simulink library "lib_wheel2"  (Simulink 10.1)
settings: Solver=VariableStepAuto  StartTime=0.0  StopTime=10.0  RelTol=1e-3
undefined symbols (not defined in the file or in its folder): lib_help, NOTES, veh_air_density, veh_CD, veh_cg_height, veh_FA, veh_front_wt_frac, veh_gravity, veh_roadwheel_radius, veh_rr_a, veh_rr_alpha, veh_rr_b, veh_rr_beta, veh_rr_c, veh_wheelbase, wh_1st_rrc, wh_2nd_rrc, wh_axle_loss_mass, wh_axle_loss_trq, wh_fa_dl_brake_frac, wh_fa_dl_brake_mph, wh_fa_fric_brake_frac, wh_fa_fric_brake_mph, wh_front_active_bool, wh_inertia, wh_max_front_brake_force, wh_max_rear_brake_force, wh_pressure, wh_radius, wh_rear_active_bool, wh_slip, wh_slip_force_coeff
undefined symbols (not defined in the file): logFlag
libraries: $bdroot x61, lib_vehicle x2, lib_etc x2, lib_controls x2, lib_wheel x1
(part 13 of 13)

== system lib_wheel2/development/wheel and axle  front/rear <wh> 2 axle --> 1 driveline/wheel & axle model & interface/wheel model/tire slip model (m/s) ==
  note: See note regarding sum in backward path
  weight borne  by front axle (N) : Inport
  total tractive  force available (N) : Inport  Port=2
  axle speed available (rad/s) : Inport  Port=3
  axle speed req'd (rad/s) : Inport  Port=4
  vehicle speed required (m/s) : Inport  Port=5
  weight borne by  rear axle (N) : Inport  Port=6
  front fraction : Inport  Port=7
  Abs1 : Abs  SaturateOnIntegerOverflow=on
  Block NOTES : Subsystem
      mask Display: disp('Block\nNOTES')
  Constant : Constant  Value=1e-3
  Constant5 : Constant
  Constant6 : Constant  Value=wh_radius
  Fcn : Fcn  Expr=1/u
  Relational Operator1 : RelationalOperator  Operator=>  RndMeth=Nearest  InputSameDT=on
  Sum1 : Sum  Inputs=+-  SaturateOnIntegerOverflow=on
  Sum2 : Sum  SaturateOnIntegerOverflow=on
  Sum3 : Sum  SaturateOnIntegerOverflow=on
  Sum4 : Sum  Inputs=-+  SaturateOnIntegerOverflow=on
  Switch1 : Switch  Threshold=eps  SaturateOnIntegerOverflow=on  InputSameDT=on
  front axle : Subsystem
  front frac : Product  SaturateOnIntegerOverflow=on
  rear axle : Subsystem
  vehicle speed (m/s) : Product  Inputs=3  SaturateOnIntegerOverflow=on
  possible vehicle speed (m/s) : Outport  InitialOutput=0
  tag scope: veh_spd_a_rec=global
  wires:
  Sum3/1 -> Fcn/1
  Fcn/1 -> vehicle speed (m/s)/1
  Constant5/1 -> Sum3/2
  axle speed available (rad/s)/1 -> Sum4/1, vehicle speed (m/s)/2
  Constant6/1 -> vehicle speed (m/s)/3
  Relational Operator1/1 -> Switch1/2
  vehicle speed required (m/s)/1 -> Switch1/3
  Sum4/1 -> Abs1/1
  axle speed req'd (rad/s)/1 -> Sum4/2
  Constant/1 -> Relational Operator1/2
  Abs1/1 -> Relational Operator1/1
  weight borne  by front axle (N)/1 -> front axle/1(In1)
  Switch1/1 -> possible vehicle speed (m/s)/1
  vehicle speed (m/s)/1 -> Switch1/1, [veh_spd_a_rec]
  weight borne by  rear axle (N)/1 -> rear axle/1(In1)
  total tractive  force available (N)/1 -> front frac/1, Sum1/1
  front fraction/1 -> front frac/2
  front frac/1 -> front axle/2(In2), Sum1/2
  Sum1/1 -> rear axle/2(In2)
  front axle/1(Out1) -> Sum2/1
  rear axle/1(Out1) -> Sum2/2
  Sum2/1 -> Sum3/1

== system lib_wheel2/development/wheel and axle  front/rear <wh> 2 axle --> 1 driveline/wheel & axle model & interface/wheel model/tire slip model (rad/s) ==
  note: Slip is defined as s=(omega*r - v) / v.  The one-to-one mapping of slip to normalized
      | tractive force, F_tract/W_front_axle, up to the maximum, is stored in the variables
      | "wh_slip" and "wh_slip_force_coeff."
  note: This block implements the effects of finite tire slip
      | (with respect to the road) on the vehicle speed/wheel speed relationship.
  note: Question: for front and rear, is it the sum of or min/max? tm:020703
  total tractive  force requested (N) : Inport
  requested time-step average vehicle speed (m/s) : Inport  Port=2
  weight borne by front axle (N) : Inport  Port=3
  weight borne by  rear axle (N)1 : Inport  Port=4
  front traction ratio : Inport  Port=5
  Constant5 : Constant
  Constant6 : Constant  Value=1/wh_radius
  Sum1 : Sum  Inputs=+-  SaturateOnIntegerOverflow=on
  Sum2 : Sum  SaturateOnIntegerOverflow=on
  Sum3 : Sum  SaturateOnIntegerOverflow=on
  To Workspace6 : ToWorkspace  VariableName=wh_slip_r  SampleTime=-1
  front frac : Product  SaturateOnIntegerOverflow=on
  front slip : Subsystem
  rear slip : Subsystem
  wheel speed (rad/s) : Product  Inputs=3  SaturateOnIntegerOverflow=on
  slip-augmented rotational speed (rad/s) : Outport  InitialOutput=0
  wires:
  weight borne by front axle (N)/1 -> front slip/1(In1)
  requested time-step average vehicle speed (m/s)/1 -> wheel speed (rad/s)/1
  Constant6/1 -> wheel speed (rad/s)/3
  Sum3/1 -> wheel speed (rad/s)/2
  Constant5/1 -> Sum3/2
  wheel speed (rad/s)/1 -> slip-augmented rotational speed (rad/s)/1
  front frac/1 -> Sum1/2, front slip/2(In2)
  total tractive  force requested (N)/1 -> front frac/1, Sum1/1
  front traction ratio/1 -> front frac/2
  Sum1/1 -> rear slip/2(In2)
  weight borne by  rear axle (N)1/1 -> rear slip/1(In1)
  front slip/1(Out1) -> Sum2/1
  rear slip/1(Out1) -> Sum2/2
  Sum2/1 -> Sum3/1, To Workspace6/1

== system lib_wheel2/development/wheel and axle  front/rear <wh> 2 axle --> 1 driveline/wheel & axle model & interface/wheel model/traction controller interface ==
  F_req : Inport
  v_ave_req : Inport  Port=2
  F_req_limited : Outport  InitialOutput=0
  v_req_limited : Outport  Port=2  InitialOutput=0
  wt_front_axle : Outport  Port=3  InitialOutput=0
  wt_rear_axle : Outport  Port=4  InitialOutput=0
  front_traction_ratio : Outport  Port=5  InitialOutput=0
  tag scope: F_req=global, v_ave_req=global
  wires:
  [F_req_limited] -> F_req_limited/1
  [v_req_limited] -> v_req_limited/1
  [wt_front_axle] -> wt_front_axle/1
  F_req/1 -> [F_req]
  v_ave_req/1 -> [v_ave_req]
  [wt_rear_axle] -> wt_rear_axle/1
  [front_traction_ratio] -> front_traction_ratio/1

== system lib_wheel2/vehicle, wheel, & axle front/rear <wh>/models and interface/vehicle <veh>/record achieved force outputs/enhancedToWorkspace ==
  In1 : Inport
  To Workspace : ToWorkspace  VariableName=veh_pwr_accel_a  SampleTime=-1
  wires:
  In1/1 -> To Workspace/1

== system lib_wheel2/vehicle, wheel, & axle front/rear <wh>/models and interface/vehicle <veh>/record achieved force outputs/enhancedToWorkspace1 ==
  In1 : Inport
  To Workspace : ToWorkspace  VariableName=veh_pwr_drag_a  SampleTime=-1
  wires:
  In1/1 -> To Workspace/1

== system lib_wheel2/vehicle, wheel, & axle front/rear <wh>/models and interface/vehicle <veh>/record achieved force outputs/enhancedToWorkspace2 ==
  In1 : Inport
  To Workspace : ToWorkspace  VariableName=veh_pwr_ascent_a  SampleTime=-1
  wires:
  In1/1 -> To Workspace/1

== system lib_wheel2/vehicle, wheel, & axle front/rear <wh>/models and interface/vehicle <veh>/record achieved force outputs/enhancedToWorkspace3 ==
  In1 : Inport
  To Workspace : ToWorkspace  VariableName=veh_pwr_rr_a  SampleTime=-1
  wires:
  In1/1 -> To Workspace/1

== system lib_wheel2/vehicle, wheel, & axle front/rear <wh>/models and interface/vehicle <veh>/record achieved force outputs/rolling resistance force ==
  average vehicle speed over time step (m/s) : Inport
  force req'd to overcome rolling resistance (N) : $bdroot/Submodels/force req'd to overcome rolling resistance (N)
      settings: RTWFcnNameOpts=Auto  RTWFileNameOpts=Auto
  Fr (N) : Outport
  wires:
  average vehicle speed over time step (m/s)/1 -> force req'd to overcome rolling resistance (N)/1
  force req'd to overcome rolling resistance (N)/1 -> Fr (N)/1

== system lib_wheel2/vehicle, wheel, & axle front/rear <wh>/models and interface/wheel and axle  front/rear <wh>/front force/brake request  controller interface ==
  F_front_brake_req : Outport  InitialOutput=0
  wires:
  [F_front_brake_req] -> F_front_brake_req/1

== system lib_wheel2/vehicle, wheel, & axle front/rear <wh>/models and interface/wheel and axle  front/rear <wh>/front force/enhancedToWorkspace11 ==
  In1 : Inport
  To Workspace : ToWorkspace  VariableName=wh_front_brake_r  SampleTime=-1
  wires:
  In1/1 -> To Workspace/1

== system lib_wheel2/vehicle, wheel, & axle front/rear <wh>/models and interface/wheel and axle  front/rear <wh>/limits and losses diagnostics/enhancedToWorkspace ==
  In1 : Inport
  To Workspace : ToWorkspace  VariableName=wh_brake_loss_pwr  SampleTime=-1
  wires:
  In1/1 -> To Workspace/1

== system lib_wheel2/vehicle, wheel, & axle front/rear <wh>/models and interface/wheel and axle  front/rear <wh>/rear force/brake request controller interface1 ==
  F_rear_brake_req : Outport  InitialOutput=0
  wires:
  [F_rear_brake_req] -> F_rear_brake_req/1

== system lib_wheel2/vehicle, wheel, & axle front/rear <wh>/models and interface/wheel and axle  front/rear <wh>/rear force/enhancedToWorkspace ==
  In1 : Inport
  To Workspace : ToWorkspace  VariableName=wh_rear_brake_r  SampleTime=-1
  wires:
  In1/1 -> To Workspace/1

== system lib_wheel2/vehicle, wheel, & axle front/rear <wh>/models and interface/wheel and axle  front/rear <wh>/tire slip model (m/s)/Block NOTES ==
  note: This block implements the effects of finite tire slip (with respect to the road) on the
      | vehicle speed/wheel speed relationship.  Slip is defined as s=(omega*r - v) / v.  The
      | one-to-one mapping of slip to normalized tractive force, F_tract/W_front_axle, up to
      | the maximum, is stored in the variables "wh_slip" and "wh_slip_force_coeff."  The
      | slip calculation here is overridden if the actual axle speed and the requested axle
      | speed are the same, indicating that no drivetrain speed limits were encountered.

== system lib_wheel2/vehicle, wheel, & axle front/rear <wh>/models and interface/wheel and axle  front/rear <wh>/tire slip model (m/s)/front axle ==
  In1 : Inport
  In2 : Inport  Port=2
  Abs : Abs  SaturateOnIntegerOverflow=on
  Constant3 : Constant  Value=0
  F/W : Product  Inputs=*/  SaturateOnIntegerOverflow=on
  Product : Product  SaturateOnIntegerOverflow=on
  Relational Operator : RelationalOperator  Operator=~=  RndMeth=Nearest  InputSameDT=on
  Saturation : Saturate  UpperLimit=max(wh_slip_force_coeff)  LowerLimit=min(wh_slip_force_coeff)
  Sign : Signum
  Switch : Switch  SaturateOnIntegerOverflow=on  InputSameDT=on
  s=s(F/W) : Lookup  InputValues=wh_slip_force_coeff  Table=wh_slip  SaturateOnIntegerOverflow=on
  Out1 : Outport
  wires:
  Constant3/1 -> Switch/3, Relational Operator/2
  Relational Operator/1 -> Switch/2
  Abs/1 -> F/W/1, Relational Operator/1
  Saturation/1 -> s=s(F/W)/1
  Switch/1 -> Saturation/1
  F/W/1 -> Switch/1
  Sign/1 -> Product/2
  s=s(F/W)/1 -> Product/1
  In2/1 -> Abs/1, Sign/1
  In1/1 -> F/W/2
  Product/1 -> Out1/1

== system lib_wheel2/vehicle, wheel, & axle front/rear <wh>/models and interface/wheel and axle  front/rear <wh>/tire slip model (m/s)/rear axle ==
  In1 : Inport
  In2 : Inport  Port=2
  Abs : Abs  SaturateOnIntegerOverflow=on
  Constant3 : Constant  Value=0
  F/W : Product  Inputs=*/  SaturateOnIntegerOverflow=on
  Product : Product  SaturateOnIntegerOverflow=on
  Relational Operator : RelationalOperator  Operator=~=  RndMeth=Nearest  InputSameDT=on
  Saturation : Saturate  UpperLimit=max(wh_slip_force_coeff)  LowerLimit=min(wh_slip_force_coeff)
  Sign : Signum
  Switch : Switch  SaturateOnIntegerOverflow=on  InputSameDT=on
  s=s(F/W) : Lookup  InputValues=wh_slip_force_coeff  Table=wh_slip  SaturateOnIntegerOverflow=on
  Out1 : Outport
  wires:
  Constant3/1 -> Switch/3, Relational Operator/2
  Relational Operator/1 -> Switch/2
  Abs/1 -> F/W/1, Relational Operator/1
  Saturation/1 -> s=s(F/W)/1
  Switch/1 -> Saturation/1
  F/W/1 -> Switch/1
  Sign/1 -> Product/2
  s=s(F/W)/1 -> Product/1
  In2/1 -> Abs/1, Sign/1
  In1/1 -> F/W/2
  Product/1 -> Out1/1

== system lib_wheel2/vehicle, wheel, & axle front/rear <wh>/models and interface/wheel and axle  front/rear <wh>/tire slip model (rad/s)/enhancedToWorkspace ==
  In1 : Inport
  To Workspace : ToWorkspace  VariableName=wh_slip_r  SampleTime=-1
  wires:
  In1/1 -> To Workspace/1

== system lib_wheel2/vehicle, wheel, & axle front/rear <wh>/models and interface/wheel and axle  front/rear <wh>/tire slip model (rad/s)/front slip ==
  In1 : Inport
  In2 : Inport  Port=2
  Abs : Abs  SaturateOnIntegerOverflow=on
  F/W : Product  Inputs=*/  SaturateOnIntegerOverflow=on
  Product : Product  SaturateOnIntegerOverflow=on
  Saturation : Saturate  UpperLimit=max(wh_slip_force_coeff)  LowerLimit=min(wh_slip_force_coeff)
  Sign : Signum
  s=s(F/W) : Lookup  InputValues=wh_slip_force_coeff  Table=wh_slip  SaturateOnIntegerOverflow=on
  Out1 : Outport
  wires:
  Saturation/1 -> s=s(F/W)/1
  F/W/1 -> Saturation/1
  Abs/1 -> F/W/1
  Sign/1 -> Product/2
  In2/1 -> Abs/1, Sign/1
  s=s(F/W)/1 -> Product/1
  In1/1 -> F/W/2
  Product/1 -> Out1/1

== system lib_wheel2/vehicle, wheel, & axle front/rear <wh>/models and interface/wheel and axle  front/rear <wh>/tire slip model (rad/s)/rear slip ==
  In1 : Inport
  In2 : Inport  Port=2
  Abs : Abs  SaturateOnIntegerOverflow=on
  F/W : Product  Inputs=*/  SaturateOnIntegerOverflow=on
  Product : Product  SaturateOnIntegerOverflow=on
  Saturation : Saturate  UpperLimit=max(wh_slip_force_coeff)  LowerLimit=min(wh_slip_force_coeff)
  Sign : Signum
  s=s(F/W) : Lookup  InputValues=wh_slip_force_coeff  Table=wh_slip  SaturateOnIntegerOverflow=on
  Out1 : Outport
  wires:
  Saturation/1 -> s=s(F/W)/1
  F/W/1 -> Saturation/1
  Abs/1 -> F/W/1
  Sign/1 -> Product/2
  In2/1 -> Abs/1, Sign/1
  s=s(F/W)/1 -> Product/1
  In1/1 -> F/W/2
  Product/1 -> Out1/1

== system lib_wheel2/vehicle, wheel, & axle front/rear <wh> 2 axle --> 1 driveline/models and interface/vehicle <veh>/power logging--achieved/Joules ==
  In1 : Inport
  To Workspace : ToWorkspace  VariableName=veh_energy_a  SampleTime=-1
  wires:
  In1/1 -> To Workspace/1

== system lib_wheel2/vehicle, wheel, & axle front/rear <wh> 2 axle --> 1 driveline/models and interface/vehicle <veh>/power logging--achieved/horse power ==
  In1 : Inport
  To Workspace : ToWorkspace  VariableName=veh_pwr_a_hp  SampleTime=-1
  wires:
  In1/1 -> To Workspace/1

== system lib_wheel2/vehicle, wheel, & axle front/rear <wh> 2 axle --> 1 driveline/models and interface/vehicle <veh>/power logging--achieved/watts ==
  In1 : Inport
  To Workspace : ToWorkspace  VariableName=veh_pwr_a  SampleTime=-1
  wires:
  In1/1 -> To Workspace/1

== system lib_wheel2/vehicle, wheel, & axle front/rear <wh> 2 axle --> 1 driveline/models and interface/vehicle <veh>/power logging--request/Joules ==
  In1 : Inport
  To Workspace : ToWorkspace  VariableName=veh_energy_r  SampleTime=-1
  wires:
  In1/1 -> To Workspace/1

== system lib_wheel2/vehicle, wheel, & axle front/rear <wh> 2 axle --> 1 driveline/models and interface/vehicle <veh>/power logging--request/horse power ==
  In1 : Inport
  To Workspace : ToWorkspace  VariableName=veh_pwr_r_hp  SampleTime=-1
  wires:
  In1/1 -> To Workspace/1

== system lib_wheel2/vehicle, wheel, & axle front/rear <wh> 2 axle --> 1 driveline/models and interface/vehicle <veh>/power logging--request/watts ==
  In1 : Inport
  To Workspace : ToWorkspace  VariableName=veh_pwr_r  SampleTime=-1
  wires:
  In1/1 -> To Workspace/1

== system lib_wheel2/vehicle, wheel, & axle front/rear <wh> 2 axle --> 1 driveline/models and interface/vehicle <veh>/record achieved force outputs/enhancedToWorkspace ==
  In1 : Inport
  To Workspace : ToWorkspace  VariableName=veh_pwr_accel_a  SampleTime=-1
  wires:
  In1/1 -> To Workspace/1

== system lib_wheel2/vehicle, wheel, & axle front/rear <wh> 2 axle --> 1 driveline/models and interface/vehicle <veh>/record achieved force outputs/enhancedToWorkspace1 ==
  In1 : Inport
  To Workspace : ToWorkspace  VariableName=veh_pwr_drag_a  SampleTime=-1
  wires:
  In1/1 -> To Workspace/1

== system lib_wheel2/vehicle, wheel, & axle front/rear <wh> 2 axle --> 1 driveline/models and interface/vehicle <veh>/record achieved force outputs/enhancedToWorkspace2 ==
  In1 : Inport
  To Workspace : ToWorkspace  VariableName=veh_pwr_ascent_a  SampleTime=-1
  wires:
  In1/1 -> To Workspace/1

== system lib_wheel2/vehicle, wheel, & axle front/rear <wh> 2 axle --> 1 driveline/models and interface/vehicle <veh>/record achieved force outputs/enhancedToWorkspace3 ==
  In1 : Inport
  To Workspace : ToWorkspace  VariableName=veh_pwr_rr_a  SampleTime=-1
  wires:
  In1/1 -> To Workspace/1

== system lib_wheel2/vehicle, wheel, & axle front/rear <wh> 2 axle --> 1 driveline/models and interface/vehicle <veh>/record achieved force outputs/rolling resistance force ==
  average vehicle speed over time step (m/s) : Inport
  force req'd to overcome rolling resistance (N) : $bdroot/Submodels/force req'd to overcome rolling resistance (N)
      settings: RTWFcnNameOpts=Auto  RTWFileNameOpts=Auto
  Fr (N) : Outport
  wires:
  force req'd to overcome rolling resistance (N)/1 -> Fr (N)/1
  average vehicle speed over time step (m/s)/1 -> force req'd to overcome rolling resistance (N)/1

== system lib_wheel2/vehicle, wheel, & axle front/rear <wh> 2 axle --> 1 driveline/models and interface/wheel and axle  front/rear <wh>/front force/brake request  controller interface ==
  F_front_brake_req : Outport  InitialOutput=0
  wires:
  [F_front_brake_req] -> F_front_brake_req/1

== system lib_wheel2/vehicle, wheel, & axle front/rear <wh> 2 axle --> 1 driveline/models and interface/wheel and axle  front/rear <wh>/front force/enhancedToWorkspace11 ==
  In1 : Inport
  To Workspace : ToWorkspace  VariableName=wh_front_brake_r  SampleTime=-1
  wires:
  In1/1 -> To Workspace/1

== system lib_wheel2/vehicle, wheel, & axle front/rear <wh> 2 axle --> 1 driveline/models and interface/wheel and axle  front/rear <wh>/limits and losses diagnostics/enhancedToWorkspace ==
  In1 : Inport
  To Workspace : ToWorkspace  VariableName=wh_brake_loss_pwr  SampleTime=-1
  wires:
  In1/1 -> To Workspace/1

== system lib_wheel2/vehicle, wheel, & axle front/rear <wh> 2 axle --> 1 driveline/models and interface/wheel and axle  front/rear <wh>/rear force/brake request controller interface1 ==
  F_rear_brake_req : Outport  InitialOutput=0
  wires:
  [F_rear_brake_req] -> F_rear_brake_req/1

== system lib_wheel2/vehicle, wheel, & axle front/rear <wh> 2 axle --> 1 driveline/models and interface/wheel and axle  front/rear <wh>/rear force/enhancedToWorkspace ==
  In1 : Inport
  To Workspace : ToWorkspace  VariableName=wh_rear_brake_r  SampleTime=-1
  wires:
  In1/1 -> To Workspace/1

== system lib_wheel2/vehicle, wheel, & axle front/rear <wh> 2 axle --> 1 driveline/models and interface/wheel and axle  front/rear <wh>/tire slip model (m/s)/Block NOTES ==
  note: This block implements the effects of finite tire slip (with respect to the road) on the
      | vehicle speed/wheel speed relationship.  Slip is defined as s=(omega*r - v) / v.  The
      | one-to-one mapping of slip to normalized tractive force, F_tract/W_front_axle, up to
      | the maximum, is stored in the variables "wh_slip" and "wh_slip_force_coeff."  The
      | slip calculation here is overridden if the actual axle speed and the requested axle
      | speed are the same, indicating that no drivetrain speed limits were encountered.

== system lib_wheel2/vehicle, wheel, & axle front/rear <wh> 2 axle --> 1 driveline/models and interface/wheel and axle  front/rear <wh>/tire slip model (m/s)/front axle ==
  In1 : Inport
  In2 : Inport  Port=2
  Abs : Abs  SaturateOnIntegerOverflow=on
  Constant3 : Constant  Value=0
  F/W : Product  Inputs=*/  SaturateOnIntegerOverflow=on
  Product : Product  SaturateOnIntegerOverflow=on
  Relational Operator : RelationalOperator  Operator=~=  RndMeth=Nearest  InputSameDT=on
  Saturation : Saturate  UpperLimit=max(wh_slip_force_coeff)  LowerLimit=min(wh_slip_force_coeff)
  Sign : Signum
  Switch : Switch  SaturateOnIntegerOverflow=on  InputSameDT=on
  s=s(F/W) : Lookup  InputValues=wh_slip_force_coeff  Table=wh_slip  SaturateOnIntegerOverflow=on
  Out1 : Outport
  wires:
  Constant3/1 -> Switch/3, Relational Operator/2
  Relational Operator/1 -> Switch/2
  Abs/1 -> F/W/1, Relational Operator/1
  Saturation/1 -> s=s(F/W)/1
  Switch/1 -> Saturation/1
  F/W/1 -> Switch/1
  Sign/1 -> Product/2
  s=s(F/W)/1 -> Product/1
  In2/1 -> Abs/1, Sign/1
  In1/1 -> F/W/2
  Product/1 -> Out1/1

== system lib_wheel2/vehicle, wheel, & axle front/rear <wh> 2 axle --> 1 driveline/models and interface/wheel and axle  front/rear <wh>/tire slip model (m/s)/rear axle ==
  In1 : Inport
  In2 : Inport  Port=2
  Abs : Abs  SaturateOnIntegerOverflow=on
  Constant3 : Constant  Value=0
  F/W : Product  Inputs=*/  SaturateOnIntegerOverflow=on
  Product : Product  SaturateOnIntegerOverflow=on
  Relational Operator : RelationalOperator  Operator=~=  RndMeth=Nearest  InputSameDT=on
  Saturation : Saturate  UpperLimit=max(wh_slip_force_coeff)  LowerLimit=min(wh_slip_force_coeff)
  Sign : Signum
  Switch : Switch  SaturateOnIntegerOverflow=on  InputSameDT=on
  s=s(F/W) : Lookup  InputValues=wh_slip_force_coeff  Table=wh_slip  SaturateOnIntegerOverflow=on
  Out1 : Outport
  wires:
  Constant3/1 -> Switch/3, Relational Operator/2
  Relational Operator/1 -> Switch/2
  Abs/1 -> F/W/1, Relational Operator/1
  Saturation/1 -> s=s(F/W)/1
  Switch/1 -> Saturation/1
  F/W/1 -> Switch/1
  Sign/1 -> Product/2
  s=s(F/W)/1 -> Product/1
  In2/1 -> Abs/1, Sign/1
  In1/1 -> F/W/2
  Product/1 -> Out1/1

== system lib_wheel2/vehicle, wheel, & axle front/rear <wh> 2 axle --> 1 driveline/models and interface/wheel and axle  front/rear <wh>/tire slip model (rad/s)/enhancedToWorkspace ==
  In1 : Inport
  To Workspace : ToWorkspace  VariableName=wh_slip_r  SampleTime=-1
  wires:
  In1/1 -> To Workspace/1

== system lib_wheel2/vehicle, wheel, & axle front/rear <wh> 2 axle --> 1 driveline/models and interface/wheel and axle  front/rear <wh>/tire slip model (rad/s)/front slip ==
  In1 : Inport
  In2 : Inport  Port=2
  Abs : Abs  SaturateOnIntegerOverflow=on
  F/W : Product  Inputs=*/  SaturateOnIntegerOverflow=on
  Product : Product  SaturateOnIntegerOverflow=on
  Saturation : Saturate  UpperLimit=max(wh_slip_force_coeff)  LowerLimit=min(wh_slip_force_coeff)
  Sign : Signum
  s=s(F/W) : Lookup  InputValues=wh_slip_force_coeff  Table=wh_slip  SaturateOnIntegerOverflow=on
  Out1 : Outport
  wires:
  Saturation/1 -> s=s(F/W)/1
  F/W/1 -> Saturation/1
  Abs/1 -> F/W/1
  Sign/1 -> Product/2
  In2/1 -> Abs/1, Sign/1
  s=s(F/W)/1 -> Product/1
  In1/1 -> F/W/2
  Product/1 -> Out1/1

== system lib_wheel2/vehicle, wheel, & axle front/rear <wh> 2 axle --> 1 driveline/models and interface/wheel and axle  front/rear <wh>/tire slip model (rad/s)/rear slip ==
  In1 : Inport
  In2 : Inport  Port=2
  Abs : Abs  SaturateOnIntegerOverflow=on
  F/W : Product  Inputs=*/  SaturateOnIntegerOverflow=on
  Product : Product  SaturateOnIntegerOverflow=on
  Saturation : Saturate  UpperLimit=max(wh_slip_force_coeff)  LowerLimit=min(wh_slip_force_coeff)
  Sign : Signum
  s=s(F/W) : Lookup  InputValues=wh_slip_force_coeff  Table=wh_slip  SaturateOnIntegerOverflow=on
  Out1 : Outport
  wires:
  Saturation/1 -> s=s(F/W)/1
  F/W/1 -> Saturation/1
  Abs/1 -> F/W/1
  Sign/1 -> Product/2
  In2/1 -> Abs/1, Sign/1
  s=s(F/W)/1 -> Product/1
  In1/1 -> F/W/2
  Product/1 -> Out1/1

== system lib_wheel2/development/wheel and axle  front/rear <wh>/wheel & axle model & interface/wheel model/front force/brake request  controller interface ==
  F_front_brake_req : Outport  InitialOutput=0
  wires:
  [F_front_brake_req] -> F_front_brake_req/1

== system lib_wheel2/development/wheel and axle  front/rear <wh>/wheel & axle model & interface/wheel model/front force/enhancedToWorkspace9 ==
  In1 : Inport
  To Workspace : ToWorkspace  VariableName=wh_front_brake_r  SampleTime=-1
  wires:
  In1/1 -> To Workspace/1

== system lib_wheel2/development/wheel and axle  front/rear <wh>/wheel & axle model & interface/wheel model/limits and losses diagnostics/enhancedToWorkspace ==
  In1 : Inport
  To Workspace : ToWorkspace  VariableName=wh_brake_loss_pwr  SampleTime=-1
  wires:
  In1/1 -> To Workspace/1

== system lib_wheel2/development/wheel and axle  front/rear <wh>/wheel & axle model & interface/wheel model/rear force/brake request controller interface1 ==
  F_rear_brake_req : Outport  InitialOutput=0
  wires:
  [F_rear_brake_req] -> F_rear_brake_req/1

== system lib_wheel2/development/wheel and axle  front/rear <wh>/wheel & axle model & interface/wheel model/rear force/enhancedToWorkspace9 ==
  In1 : Inport
  To Workspace : ToWorkspace  VariableName=wh_rear_brake_r  SampleTime=-1
  wires:
  In1/1 -> To Workspace/1

== system lib_wheel2/development/wheel and axle  front/rear <wh>/wheel & axle model & interface/wheel model/rolling resistance add/Rolling Resistance Force (N) ==
  In1 : Inport
  To Workspace : ToWorkspace  VariableName=wh_Fr  SampleTime=-1
  wires:
  In1/1 -> To Workspace/1

== system lib_wheel2/development/wheel and axle  front/rear <wh>/wheel & axle model & interface/wheel model/rolling resistance add/enhancedToWorkspace3 ==
  In1 : Inport
  To Workspace : ToWorkspace  VariableName=wh_force_r  SampleTime=-1
  wires:
  In1/1 -> To Workspace/1

== system lib_wheel2/development/wheel and axle  front/rear <wh>/wheel & axle model & interface/wheel model/rolling resistance add/rolling resistance force ==
  average vehicle speed over time step (m/s) : Inport
  force req'd to overcome rolling resistance (N) : $bdroot/Submodels/force req'd to overcome rolling resistance (N)
      settings: RTWFcnNameOpts=Auto  RTWFileNameOpts=Auto
  Fr (N) : Outport
  wires:
  average vehicle speed over time step (m/s)/1 -> force req'd to overcome rolling resistance (N)/1
  force req'd to overcome rolling resistance (N)/1 -> Fr (N)/1

== system lib_wheel2/development/wheel and axle  front/rear <wh>/wheel & axle model & interface/wheel model/rolling resistance deduct/Rolling Resistance Force (N) ==
  In1 : Inport
  To Workspace : ToWorkspace  VariableName=wh_Fr_ach  SampleTime=-1
  wires:
  In1/1 -> To Workspace/1

== system lib_wheel2/development/wheel and axle  front/rear <wh>/wheel & axle model & interface/wheel model/rolling resistance deduct/enhancedToWorkspace3 ==
  In1 : Inport
  To Workspace : ToWorkspace  VariableName=wh_force_a  SampleTime=-1
  wires:
  In1/1 -> To Workspace/1

== system lib_wheel2/development/wheel and axle  front/rear <wh>/wheel & axle model & interface/wheel model/rolling resistance deduct/rolling resistance force ==
  average vehicle speed over time step (m/s) : Inport
  force req'd to overcome rolling resistance (N) : $bdroot/Submodels/force req'd to overcome rolling resistance (N)
      settings: RTWFcnNameOpts=Auto  RTWFileNameOpts=Auto
  Fr (N) : Outport
  wires:
  average vehicle speed over time step (m/s)/1 -> force req'd to overcome rolling resistance (N)/1
  force req'd to overcome rolling resistance (N)/1 -> Fr (N)/1

== system lib_wheel2/development/wheel and axle  front/rear <wh>/wheel & axle model & interface/wheel model/tire slip model (m/s)/Block NOTES ==
  note: This block implements the effects of finite tire slip (with respect to the road) on the
      | vehicle speed/wheel speed relationship.  Slip is defined as s=(omega*r - v) / v.  The
      | one-to-one mapping of slip to normalized tractive force, F_tract/W_front_axle, up to
      | the maximum, is stored in the variables "wh_slip" and "wh_slip_force_coeff."  The
      | slip calculation here is overridden if the actual axle speed and the requested axle
      | speed are the same, indicating that no drivetrain speed limits were encountered.

== system lib_wheel2/development/wheel and axle  front/rear <wh>/wheel & axle model & interface/wheel model/tire slip model (m/s)/front axle ==
  In1 : Inport
  In2 : Inport  Port=2
  Abs : Abs  SaturateOnIntegerOverflow=on
  Constant3 : Constant  Value=0
  F/W : Product  Inputs=*/  SaturateOnIntegerOverflow=on
  Product : Product  SaturateOnIntegerOverflow=on
  Relational Operator : RelationalOperator  Operator=~=  RndMeth=Nearest  InputSameDT=on
  Saturation : Saturate  UpperLimit=max(wh_slip_force_coeff)  LowerLimit=min(wh_slip_force_coeff)
  Sign : Signum
  Switch : Switch  SaturateOnIntegerOverflow=on  InputSameDT=on
  s=s(F/W) : Lookup  InputValues=wh_slip_force_coeff  Table=wh_slip  SaturateOnIntegerOverflow=on
  Out1 : Outport
  wires:
  Constant3/1 -> Switch/3, Relational Operator/2
  Relational Operator/1 -> Switch/2
  Abs/1 -> F/W/1, Relational Operator/1
  Saturation/1 -> s=s(F/W)/1
  Switch/1 -> Saturation/1
  F/W/1 -> Switch/1
  Sign/1 -> Product/2
  s=s(F/W)/1 -> Product/1
  In2/1 -> Abs/1, Sign/1
  In1/1 -> F/W/2
  Product/1 -> Out1/1

== system lib_wheel2/development/wheel and axle  front/rear <wh>/wheel & axle model & interface/wheel model/tire slip model (m/s)/rear axle ==
  In1 : Inport
  In2 : Inport  Port=2
  Abs : Abs  SaturateOnIntegerOverflow=on
  Constant3 : Constant  Value=0
  F/W : Product  Inputs=*/  SaturateOnIntegerOverflow=on
  Product : Product  SaturateOnIntegerOverflow=on
  Relational Operator : RelationalOperator  Operator=~=  RndMeth=Nearest  InputSameDT=on
  Saturation : Saturate  UpperLimit=max(wh_slip_force_coeff)  LowerLimit=min(wh_slip_force_coeff)
  Sign : Signum
  Switch : Switch  SaturateOnIntegerOverflow=on  InputSameDT=on
  s=s(F/W) : Lookup  InputValues=wh_slip_force_coeff  Table=wh_slip  SaturateOnIntegerOverflow=on
  Out1 : Outport
  wires:
  Constant3/1 -> Switch/3, Relational Operator/2
  Relational Operator/1 -> Switch/2
  Abs/1 -> F/W/1, Relational Operator/1
  Saturation/1 -> s=s(F/W)/1
  Switch/1 -> Saturation/1
  F/W/1 -> Switch/1
  Sign/1 -> Product/2
  s=s(F/W)/1 -> Product/1
  In2/1 -> Abs/1, Sign/1
  In1/1 -> F/W/2
  Product/1 -> Out1/1

== system lib_wheel2/development/wheel and axle  front/rear <wh>/wheel & axle model & interface/wheel model/tire slip model (rad/s)/enhancedToWorkspace9 ==
  In1 : Inport
  To Workspace : ToWorkspace  VariableName=wh_slip_r  SampleTime=-1
  wires:
  In1/1 -> To Workspace/1

== system lib_wheel2/development/wheel and axle  front/rear <wh>/wheel & axle model & interface/wheel model/tire slip model (rad/s)/front slip ==
  In1 : Inport
  In2 : Inport  Port=2
  Abs : Abs  SaturateOnIntegerOverflow=on
  F/W : Product  Inputs=*/  SaturateOnIntegerOverflow=on
  Product : Product  SaturateOnIntegerOverflow=on
  Saturation : Saturate  UpperLimit=max(wh_slip_force_coeff)  LowerLimit=min(wh_slip_force_coeff)
  Sign : Signum
  s=s(F/W) : Lookup  InputValues=wh_slip_force_coeff  Table=wh_slip  SaturateOnIntegerOverflow=on
  Out1 : Outport
  wires:
  Saturation/1 -> s=s(F/W)/1
  F/W/1 -> Saturation/1
  Abs/1 -> F/W/1
  Sign/1 -> Product/2
  In2/1 -> Abs/1, Sign/1
  s=s(F/W)/1 -> Product/1
  In1/1 -> F/W/2
  Product/1 -> Out1/1

== system lib_wheel2/development/wheel and axle  front/rear <wh>/wheel & axle model & interface/wheel model/tire slip model (rad/s)/rear slip ==
  In1 : Inport
  In2 : Inport  Port=2
  Abs : Abs  SaturateOnIntegerOverflow=on
  F/W : Product  Inputs=*/  SaturateOnIntegerOverflow=on
  Product : Product  SaturateOnIntegerOverflow=on
  Saturation : Saturate  UpperLimit=max(wh_slip_force_coeff)  LowerLimit=min(wh_slip_force_coeff)
  Sign : Signum
  s=s(F/W) : Lookup  InputValues=wh_slip_force_coeff  Table=wh_slip  SaturateOnIntegerOverflow=on
  Out1 : Outport
  wires:
  Saturation/1 -> s=s(F/W)/1
  F/W/1 -> Saturation/1
  Abs/1 -> F/W/1
  Sign/1 -> Product/2
  In2/1 -> Abs/1, Sign/1
  s=s(F/W)/1 -> Product/1
  In1/1 -> F/W/2
  Product/1 -> Out1/1

== system lib_wheel2/development/wheel and axle  front/rear <wh>/wheel & axle model & interface/wheel model/traction controller interface/config traction control ==
  time-average vehicle speed  req'd (m/s) : Inport
  vehicle speed at beginning of time  step (m/s) : Inport  Port=2
  total tractive force req'd (N) : Inport  Port=3
  traction control 2 axle : $bdroot/Submodels/traction control 2 axle
      settings: RTWFcnNameOpts=Auto  RTWFileNameOpts=Auto
  req'd force (N) : Outport
  req'd speed (m/s) : Outport  Port=2
  weight on front axle (N) : Outport  Port=3
  weight on rear axle (N) : Outport  Port=4
  front/total  traction ratio : Outport  Port=5
  wires:
  time-average vehicle speed  req'd (m/s)/1 -> traction control 2 axle/1
  vehicle speed at beginning of time  step (m/s)/1 -> traction control 2 axle/2
  total tractive force req'd (N)/1 -> traction control 2 axle/3
  traction control 2 axle/1 -> req'd force (N)/1
  traction control 2 axle/2 -> req'd speed (m/s)/1
  traction control 2 axle/3 -> weight on front axle (N)/1
  traction control 2 axle/4 -> weight on rear axle (N)/1
  traction control 2 axle/5 -> front/total  traction ratio/1

== system lib_wheel2/development/wheel and axle  front/rear <wh>/wheel & axle model & interface/wheel model/traction controller interface/front and rear brake controller (achievable) ==
  total tractive force req'd (N) : Inport
  tractive force available from  front drivetrain (N) : Inport  Port=2
  axle speed possible (rad/s) : Inport  Port=3
  max front brake force (N) : Inport  Port=4
  max rear brake force (N) : Inport  Port=5
  tractive force available from  rear drivetrain (N) : Inport  Port=6
  Block NOTES : lib_controls/SubSystem/front and rear brake controller (achievable)/Block NOTES
  Constant : Constant  Value=0
  Constant1 : Constant  Value=0
  MinMax : MinMax  Inputs=2
  MinMax1 : MinMax  Inputs=2
  MinMax2 : MinMax  Function=max  Inputs=2
  Sum1 : Sum  Inputs=+--  SaturateOnIntegerOverflow=on
  Sum2 : Sum  Inputs=+-  SaturateOnIntegerOverflow=on
  Switch: braking force to be split between friction brakes (N) : Switch  SaturateOnIntegerOverflow=on  InputSameDT=on
  braking force supplied by front friction brakes (N) : lib_controls/SubSystem/front and rear brake controller (achievable)/braking force supplied by front friction brakes (N)
      settings: RTWFcnNameOpts=Auto  RTWFileNameOpts=Auto
  "m/s -> mph (mph)" : Gain  Gain=2.237  SaturateOnIntegerOverflow=on
  "rad/s -> m/s (m/s)" : Gain  Gain=wh_radius  SaturateOnIntegerOverflow=on
  rear braking force req'd (N) : Switch  SaturateOnIntegerOverflow=on  InputSameDT=on
  front-axle braking force (N) : Outport  InitialOutput=0
  rear-axle braking force (N) : Outport  Port=2  InitialOutput=0
  wires:
  tractive force available from  rear drivetrain (N)/1 -> Sum1/3
  braking force supplied by front friction brakes (N)/1 -> front-axle braking force (N)/1, Sum2/2
  Switch: braking force to be split between friction brakes (N)/1 -> Sum2/1, rear braking force req'd (N)/2, braking force supplied by front friction brakes (N)/1
  "m/s -> mph (mph)"/1 -> braking force supplied by front friction brakes (N)/2
  Constant/1 -> MinMax1/1, Switch: braking force to be split between friction brakes (N)/1
  MinMax1/1 -> Switch: braking force to be split between friction brakes (N)/3
  Sum1/1 -> MinMax1/2
  total tractive force req'd (N)/1 -> Switch: braking force to be split between friction brakes (N)/2, Sum1/1
  tractive force available from  front drivetrain (N)/1 -> Sum1/2
  axle speed possible (rad/s)/1 -> "rad/s -> m/s (m/s)"/1
  "rad/s -> m/s (m/s)"/1 -> "m/s -> mph (mph)"/1
  MinMax2/1 -> rear-axle braking force (N)/1
  rear braking force req'd (N)/1 -> MinMax2/1
  Sum2/1 -> MinMax/2
  MinMax/1 -> rear braking force req'd (N)/3
  Constant1/1 -> MinMax/1, rear braking force req'd (N)/1
  max front brake force (N)/1 -> braking force supplied by front friction brakes (N)/3
  max rear brake force (N)/1 -> MinMax2/2

== system lib_wheel2/development/wheel and axle  front/rear <wh> 2 axle --> 1 driveline/wheel & axle model & interface/wheel model/front force/brake request  controller interface ==
  F_front_brake_req : Outport  InitialOutput=0
  wires:
  [F_front_brake_req] -> F_front_brake_req/1

== system lib_wheel2/development/wheel and axle  front/rear <wh> 2 axle --> 1 driveline/wheel & axle model & interface/wheel model/rear force/brake request controller interface1 ==
  F_rear_brake_req : Outport  InitialOutput=0
  wires:
  [F_rear_brake_req] -> F_rear_brake_req/1

== system lib_wheel2/development/wheel and axle  front/rear <wh> 2 axle --> 1 driveline/wheel & axle model & interface/wheel model/tire slip model (m/s)/Block NOTES ==
  note: This block implements the effects of finite tire slip (with respect to the road) on the
      | vehicle speed/wheel speed relationship.  Slip is defined as s=(omega*r - v) / v.  The
      | one-to-one mapping of slip to normalized tractive force, F_tract/W_front_axle, up to
      | the maximum, is stored in the variables "wh_slip" and "wh_slip_force_coeff."  The
      | slip calculation here is overridden if the actual axle speed and the requested axle
      | speed are the same, indicating that no drivetrain speed limits were encountered.

== system lib_wheel2/development/wheel and axle  front/rear <wh> 2 axle --> 1 driveline/wheel & axle model & interface/wheel model/tire slip model (m/s)/front axle ==
  In1 : Inport
  In2 : Inport  Port=2
  Abs : Abs  SaturateOnIntegerOverflow=on
  Constant3 : Constant  Value=0
  F/W : Product  Inputs=*/  SaturateOnIntegerOverflow=on
  Product : Product  SaturateOnIntegerOverflow=on
  Relational Operator : RelationalOperator  Operator=~=  RndMeth=Nearest  InputSameDT=on
  Saturation : Saturate  UpperLimit=max(wh_slip_force_coeff)  LowerLimit=min(wh_slip_force_coeff)
  Sign : Signum
  Switch : Switch  SaturateOnIntegerOverflow=on  InputSameDT=on
  s=s(F/W) : Lookup  InputValues=wh_slip_force_coeff  Table=wh_slip  SaturateOnIntegerOverflow=on
  Out1 : Outport
  wires:
  Constant3/1 -> Switch/3, Relational Operator/2
  Relational Operator/1 -> Switch/2
  Abs/1 -> F/W/1, Relational Operator/1
  Saturation/1 -> s=s(F/W)/1
  Switch/1 -> Saturation/1
  F/W/1 -> Switch/1
  Sign/1 -> Product/2
  s=s(F/W)/1 -> Product/1
  In2/1 -> Abs/1, Sign/1
  In1/1 -> F/W/2
  Product/1 -> Out1/1

== system lib_wheel2/development/wheel and axle  front/rear <wh> 2 axle --> 1 driveline/wheel & axle model & interface/wheel model/tire slip model (m/s)/rear axle ==
  In1 : Inport
  In2 : Inport  Port=2
  Abs : Abs  SaturateOnIntegerOverflow=on
  Constant3 : Constant  Value=0
  F/W : Product  Inputs=*/  SaturateOnIntegerOverflow=on
  Product : Product  SaturateOnIntegerOverflow=on
  Relational Operator : RelationalOperator  Operator=~=  RndMeth=Nearest  InputSameDT=on
  Saturation : Saturate  UpperLimit=max(wh_slip_force_coeff)  LowerLimit=min(wh_slip_force_coeff)
  Sign : Signum
  Switch : Switch  SaturateOnIntegerOverflow=on  InputSameDT=on
  s=s(F/W) : Lookup  InputValues=wh_slip_force_coeff  Table=wh_slip  SaturateOnIntegerOverflow=on
  Out1 : Outport
  wires:
  Constant3/1 -> Switch/3, Relational Operator/2
  Relational Operator/1 -> Switch/2
  Abs/1 -> F/W/1, Relational Operator/1
  Saturation/1 -> s=s(F/W)/1
  Switch/1 -> Saturation/1
  F/W/1 -> Switch/1
  Sign/1 -> Product/2
  s=s(F/W)/1 -> Product/1
  In2/1 -> Abs/1, Sign/1
  In1/1 -> F/W/2
  Product/1 -> Out1/1

== system lib_wheel2/development/wheel and axle  front/rear <wh> 2 axle --> 1 driveline/wheel & axle model & interface/wheel model/tire slip model (rad/s)/front slip ==
  In1 : Inport
  In2 : Inport  Port=2
  Abs : Abs  SaturateOnIntegerOverflow=on
  F/W : Product  Inputs=*/  SaturateOnIntegerOverflow=on
  Product : Product  SaturateOnIntegerOverflow=on
  Saturation : Saturate  UpperLimit=max(wh_slip_force_coeff)  LowerLimit=min(wh_slip_force_coeff)
  Sign : Signum
  s=s(F/W) : Lookup  InputValues=wh_slip_force_coeff  Table=wh_slip  SaturateOnIntegerOverflow=on
  Out1 : Outport
  wires:
  Saturation/1 -> s=s(F/W)/1
  F/W/1 -> Saturation/1
  Abs/1 -> F/W/1
  Sign/1 -> Product/2
  In2/1 -> Abs/1, Sign/1
  s=s(F/W)/1 -> Product/1
  In1/1 -> F/W/2
  Product/1 -> Out1/1

== system lib_wheel2/development/wheel and axle  front/rear <wh> 2 axle --> 1 driveline/wheel & axle model & interface/wheel model/tire slip model (rad/s)/rear slip ==
  In1 : Inport
  In2 : Inport  Port=2
  Abs : Abs  SaturateOnIntegerOverflow=on
  F/W : Product  Inputs=*/  SaturateOnIntegerOverflow=on
  Product : Product  SaturateOnIntegerOverflow=on
  Saturation : Saturate  UpperLimit=max(wh_slip_force_coeff)  LowerLimit=min(wh_slip_force_coeff)
  Sign : Signum
  s=s(F/W) : Lookup  InputValues=wh_slip_force_coeff  Table=wh_slip  SaturateOnIntegerOverflow=on
  Out1 : Outport
  wires:
  Saturation/1 -> s=s(F/W)/1
  F/W/1 -> Saturation/1
  Abs/1 -> F/W/1
  Sign/1 -> Product/2
  In2/1 -> Abs/1, Sign/1
  s=s(F/W)/1 -> Product/1
  In1/1 -> F/W/2
  Product/1 -> Out1/1
